simulink model "Transmitter"  (R2021b)
settings: Solver=VariableStepAuto  StartTime=0.0  StopTime=10.0  RelTol=1e-3
libraries: dsparch4 x2, commrandsrc3 x2, commutil2 x2, commchan3 x1
settings Model: Creator=moha  LastModifiedBy=moha

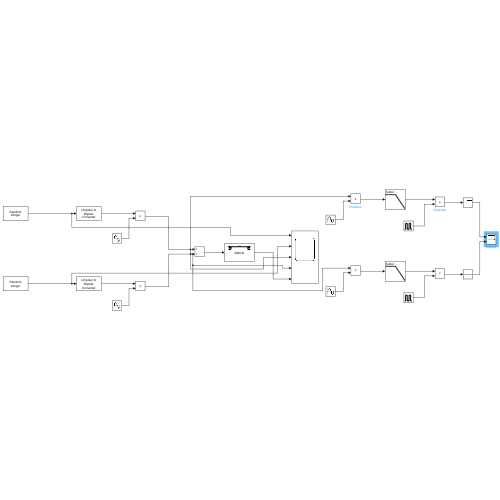
[thumbnail: Simulink's stored preview of the top-level diagram]
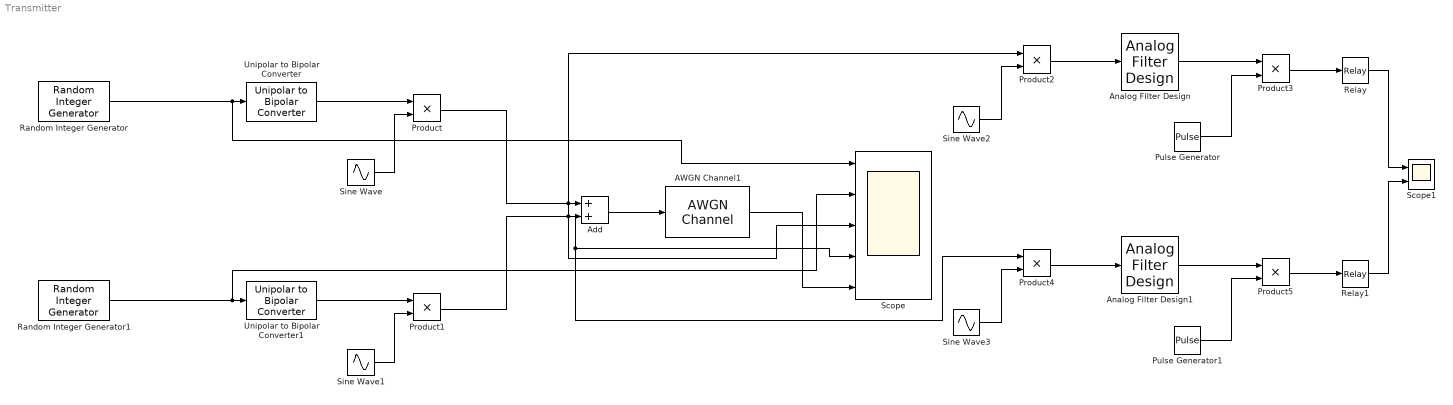
== system Transmitter ==
  AWGN Channel1 : commchan3/AWGN Channel  InputProcessing=Columns as channels (frame based)  seed=67  noiseMode="Signal to noise ratio  (SNR)"  EbNodB=10  EsNodB=10  SNRdB=50  bitsPerSym=1  Ps=1  Tsym=1  variance=1
  Add : Sum
  Analog Filter Design : dsparch4/Analog Filter Design  method=Butterworth  filttype=Lowpass  N=16  Wlo=25  Whi=80  Rp=2  Rs=40
  Analog Filter Design1 : dsparch4/Analog Filter Design  method=Butterworth  filttype=Lowpass  N=16  Wlo=25  Whi=80  Rp=2  Rs=40
  Product{,1..5} (6 alike) : Product
  Pulse Generator : DiscretePulseGenerator  PulseType=Time based  Period=0.2  PulseWidth=0.1
  Pulse Generator1 : DiscretePulseGenerator  PulseType=Time based  Period=0.2  PulseWidth=0.1
  Random Integer Generator : commrandsrc3/Random Integer Generator  SetSize=2  SeedSource=Auto  Seed=0  SampleTime=1  SamplesPerFrame=1  OutputDataType=double  SimulateUsing=Interpreted execution
  Random Integer Generator1 : commrandsrc3/Random Integer Generator  SetSize=2  SeedSource=Auto  Seed=0  SampleTime=1  SamplesPerFrame=1  OutputDataType=double  SimulateUsing=Interpreted execution
  Relay : Relay  OnSwitchValue=0.1  OffSwitchValue=-0.1
  Relay1 : Relay  OnSwitchValue=0.1  OffSwitchValue=-0.1
  Scope : Scope  NumInputPorts=5
  Scope1 : Scope  NumInputPorts=2
  Sine Wave : Sin  Frequency=20  SampleTime=0.01
  Sine Wave1 : Sin  Frequency=20  Phase=pi/2  SampleTime=0.01
  Sine Wave2 : Sin  Frequency=20  SampleTime=0.01
  Sine Wave3 : Sin  Frequency=20  Phase=pi/2  SampleTime=0.01
  Unipolar to Bipolar Converter : commutil2/Unipolar to Bipolar Converter  M=2  polarity=Positive  dataType=Inherit via internal rule
  Unipolar to Bipolar Converter1 : commutil2/Unipolar to Bipolar Converter  M=2  polarity=Positive  dataType=Inherit via internal rule
  wires:
  Unipolar to Bipolar Converter/1 -> Product/1
  Sine Wave/1 -> Product/2
  Unipolar to Bipolar Converter1/1 -> Product1/1
  Sine Wave1/1 -> Product1/2
  Product/1 -> Scope/3, Add/1, Product2/1
  Product1/1 -> Scope/4, Product4/1, Add/2
  Random Integer Generator1/1 -> Scope/2, Unipolar to Bipolar Converter1/1
  Add/1 -> AWGN Channel1/1
  AWGN Channel1/1 -> Scope/5
  Random Integer Generator/1 -> Scope/1, Unipolar to Bipolar Converter/1
  Sine Wave2/1 -> Product2/2
  Product2/1 -> Analog Filter Design/1
  Analog Filter Design/1 -> Product3/1
  Pulse Generator/1 -> Product3/2
  Product3/1 -> Relay/1
  Pulse Generator1/1 -> Product5/2
  Analog Filter Design1/1 -> Product5/1
  Product4/1 -> Analog Filter Design1/1
  Product5/1 -> Relay1/1
  Sine Wave3/1 -> Product4/2
  Relay/1 -> Scope1/1
  Relay1/1 -> Scope1/2
